simulink library "csu_mct_microcontroller_timer_sim_lib"  (R2014b)
settings: Solver=ode45  StartTime=0.0  StopTime=10.0  RelTol=1e-3
undefined symbols (not defined in the file): fsw_dt, sim_time_step_size
libraries: simulink x4, util_common_lib x2, util_info_lib x1
settings Model: Creator=escrane  LastModifiedBy=mstewart

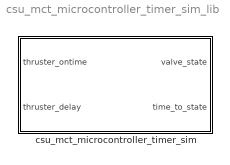
== system csu_mct_microcontroller_timer_sim_lib ==
  csu_mct_microcontroller_timer_sim : Subsystem

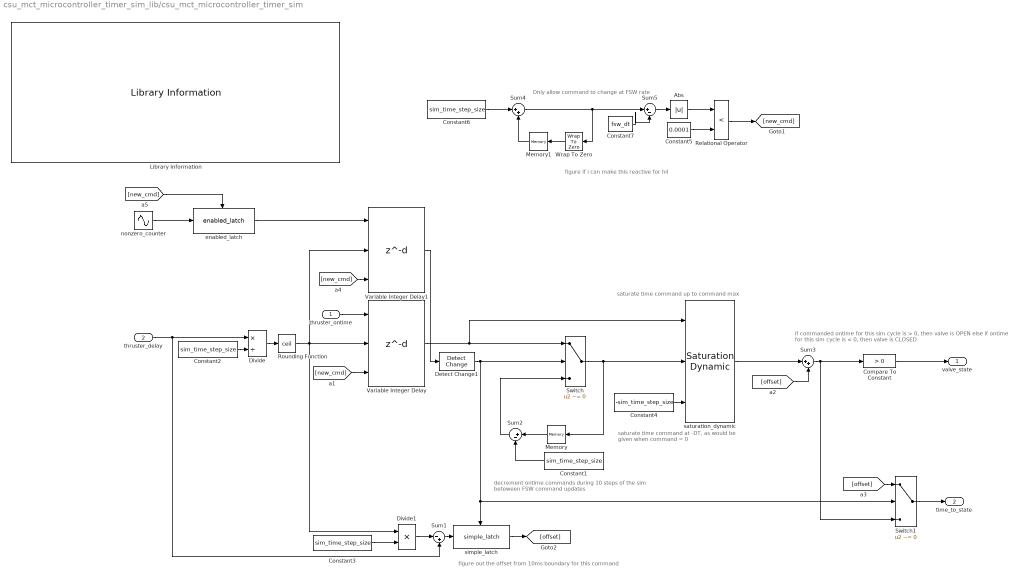
== system csu_mct_microcontroller_timer_sim_lib/csu_mct_microcontroller_timer_sim ==
  note: Only allow command to change at FSW rate
  note: decrement ontime commands during 10 steps of the
      | sim beteween FSW command updates
  note: saturate time command up to command max
  note: saturate time command at -DT,
      | as would be given when command = 0
  note: if commanded ontime for this sim cycle is > 0, then valve is OPEN
      | else if ontime for this sim cycle  is < 0, then valve is CLOSED
  note: figure out the offset from 10ms boundary for this command
  note: figure if i can make this reactive for hil
  thruster_ontime : Inport
  thruster_delay : Inport  Port=2
  Abs : Abs
  Compare To Constant : simulink/Logic and Bit Operations/Compare To Constant  relop=>  const=0  OutDataTypeStr=boolean
  Constant1 : Constant  Value=sim_time_step_size
  Constant2 : Constant  Value=sim_time_step_size
  Constant3 : Constant  Value=sim_time_step_size
  Constant4 : Constant  Value=-sim_time_step_size
  Constant5 : Constant  Value=0.0001  OutDataTypeStr=double
  Constant6 : Constant  Value=sim_time_step_size  OutDataTypeStr=double
  Constant7 : Constant  Value=fsw_dt  OutDataTypeStr=double
  Detect Change1 : simulink/Logic and Bit Operations/Detect Change  vinit=0  InputProcessing=Inherited  OutDataTypeStr=boolean
  Divide : Product  Inputs=*/
  Divide1 : Product  Inputs=**
  Library Information : util_info_lib/Library Information  owner='escrane'
  Memory : Memory  InheritSampleTime=on
  Memory1 : Memory  X0=fsw_dt - sim_time_step_size  InheritSampleTime=on
  Relational Operator : RelationalOperator  Operator=<  OutDataTypeStr=boolean
  Rounding Function : Rounding  Operator=ceil
  Sum1 : Sum  Inputs=|-+
  Sum2 : Sum  Inputs=|+-
  Sum3 : Sum  Inputs=|++
  Sum4 : Sum  Inputs=|++
  Sum5 : Sum  Inputs=|+-
  Switch : Switch  Criteria=u2 ~= 0  Threshold=0.5
  Switch1 : Switch  Criteria=u2 ~= 0  Threshold=0.5
  Variable Integer Delay : Delay  DelayLengthSource=Input port  ExternalReset=Rising
      settings: InputPortMap=u0,p1,r5
  Variable Integer Delay1 : Delay  DelayLengthSource=Input port  ExternalReset=Rising
      settings: InputPortMap=u0,p1,r5
  Wrap To Zero : simulink/Discontinuities/Wrap To Zero  Threshold=fsw_dt*.99
  enabled_latch : util_common_lib/enabled_latch  initial_output=1
  nonzero_counter : Sin  Bias=10  SampleTime=sim_time_step_size
  saturation_dynamic : simulink/Discontinuities/Saturation Dynamic  OutMin=[]  OutMax=[]  OutDataTypeStr=Inherit: Same as second input  OutDataType=fixdt(1, 16)  OutScaling=2^-10  DoSatur=off
  simple_latch : util_common_lib/simple_latch  SystemSampleTime=-1
  valve_state : Outport
  time_to_state : Outport  Port=2
  wires:
  Variable Integer Delay1/1 -> Detect Change1/1
  enabled_latch/1 -> Variable Integer Delay1/1
  [new_cmd] -> enabled_latch/Enable
  nonzero_counter/1 -> enabled_latch/1
  [new_cmd] -> Variable Integer Delay1/3
  Relational Operator/1 -> [new_cmd]
  Constant5/1 -> Relational Operator/2
  Abs/1 -> Relational Operator/1
  Sum5/1 -> Abs/1
  Constant7/1 -> Sum5/2
  Constant6/1 -> Sum4/1
  Memory1/1 -> Sum4/2
  Wrap To Zero/1 -> Memory1/1
  Sum4/1 -> Sum5/1, Wrap To Zero/1
  [offset] -> Sum3/2
  simple_latch/1 -> [offset]
  [offset] -> Switch1/1
  Divide1/1 -> Sum1/1
  Constant3/1 -> Divide1/2
  Sum3/1 -> Compare To Constant/1, Switch1/3
  Switch1/1 -> time_to_state/1
  Sum1/1 -> simple_latch/1
  Detect Change1/1 -> simple_latch/Trigger, Switch1/2, Switch/2
  saturation_dynamic/1 -> Sum3/1
  Variable Integer Delay/1 -> Switch/1, saturation_dynamic/1
  [new_cmd] -> Variable Integer Delay/3
  Rounding Function/1 -> Variable Integer Delay/2, Divide1/1, Variable Integer Delay1/2
  Divide/1 -> Rounding Function/1
  Constant2/1 -> Divide/2
  thruster_delay/1 -> Divide/1, Sum1/2
  Memory/1 -> Sum2/1
  Switch/1 -> saturation_dynamic/2, Memory/1
  Sum2/1 -> Switch/3
  Constant4/1 -> saturation_dynamic/3
  Constant1/1 -> Sum2/2
  thruster_ontime/1 -> Variable Integer Delay/1
  Compare To Constant/1 -> valve_state/1
